simulink model "Geometric_DMP_R2022a"  (R2022a)
settings: Solver=FixedStepDiscrete  StartTime=0.0  StopTime=T  FixedStep=Ts  RelTol=1e-3
undefined symbols (not defined in the file): a, b, DiscIntNeverNeededParam, eta, gd, gr, Ts, yd
libraries: simulink x2
settings Model: Creator=giovanni  LastModifiedBy=giovanni

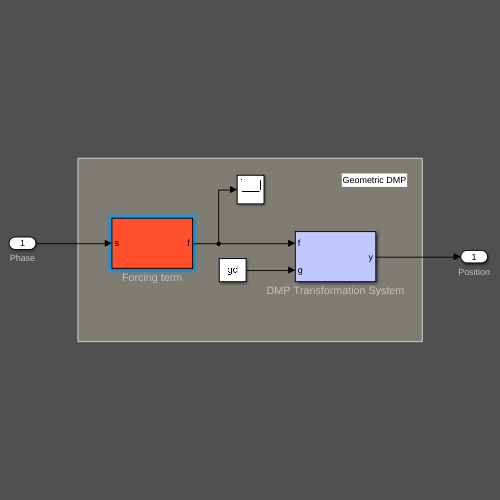
[thumbnail: Simulink's stored preview of the top-level diagram]
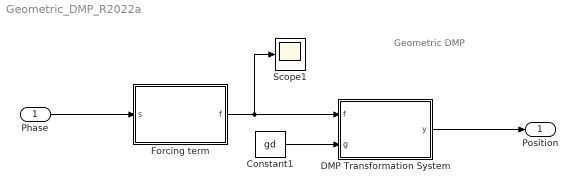
== system Geometric_DMP_R2022a ==
  note: Geometric DMP
  Phase : Inport
  Constant1 : Constant  Value=gd
  DMP Transformation System : Subsystem
  Forcing term : Subsystem
  Scope1 : Scope
  Position : Outport
  wires:
  Forcing term/1(f) -> Scope1/1, DMP Transformation System/1(f)
  Constant1/1 -> DMP Transformation System/2(g)
  DMP Transformation System/1(y) -> Position/1
  Phase/1 -> Forcing term/1(s)

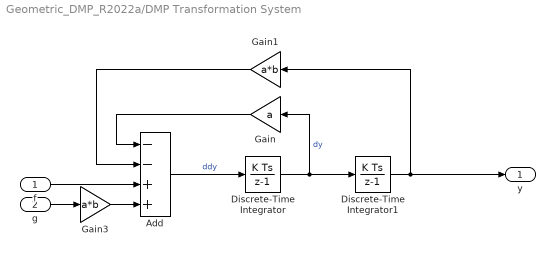
== system Geometric_DMP_R2022a/DMP Transformation System ==
  f : Inport
  g : Inport  Port=2
  Add : Sum  Inputs=--++
  Discrete-Time Integrator : DiscreteIntegrator  SampleTime=-1  ICPrevOutput=DiscIntNeverNeededParam  ICPrevScaledInput=DiscIntNeverNeededParam
  Discrete-Time Integrator1 : DiscreteIntegrator  InitialCondition=yd  SampleTime=-1  ICPrevOutput=DiscIntNeverNeededParam  ICPrevScaledInput=DiscIntNeverNeededParam
  Gain : Gain  Gain=a
  Gain1 : Gain  Gain=a*b
  Gain3 : Gain  Gain=a*b
  y : Outport
  wires:
  g/1 -> Gain3/1
  Discrete-Time Integrator/1 -> Gain/1, Discrete-Time Integrator1/1  "dy"
  Discrete-Time Integrator1/1 -> Gain1/1, y/1
  Add/1 -> Discrete-Time Integrator/1  "ddy"
  f/1 -> Add/3
  Gain/1 -> Add/1
  Gain1/1 -> Add/2
  Gain3/1 -> Add/4

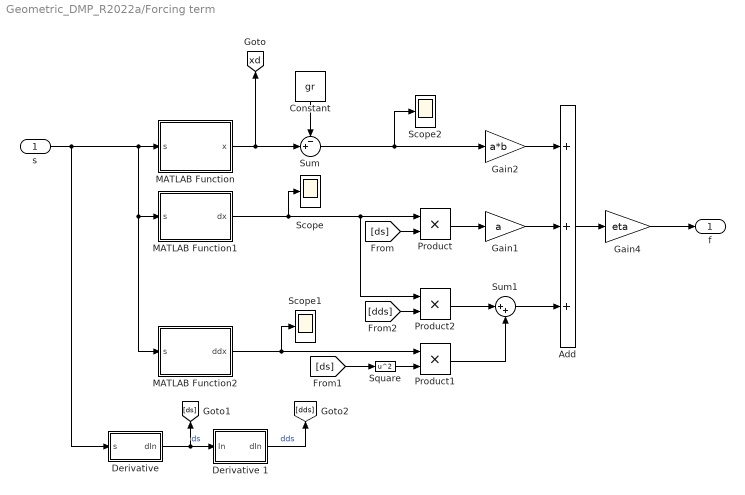
== system Geometric_DMP_R2022a/Forcing term ==
  s : Inport
  Add : Sum  Inputs=+++
  Constant : Constant  Value=gr
  "Derivative " : Subsystem
  Derivative 1 : Subsystem
  Gain1 : Gain  Gain=a
  Gain2 : Gain  Gain=a*b
  Gain4 : Gain  Gain=eta
  MATLAB Function : MATLAB Function  TreatAsAtomicUnit=on
  MATLAB Function1 : MATLAB Function  TreatAsAtomicUnit=on
  MATLAB Function2 : MATLAB Function  TreatAsAtomicUnit=on
  Product : Product
  Product1 : Product
  Product2 : Product
  Scope : Scope
  Scope1 : Scope
  Scope2 : Scope
  Square : Math  Operator=square
  Sum : Sum  Inputs=-+|
  Sum1 : Sum  Inputs=|++
  f : Outport
  tag scope: xd=global
  wires:
  s/1 -> "Derivative "/1(s), MATLAB Function2/1(s), MATLAB Function1/1(s), MATLAB Function/1(s)
  MATLAB Function/1(x) -> Sum/2, [xd]
  Constant/1 -> Sum/1
  MATLAB Function1/1(dx) -> Product2/1, Product/1, Scope/1
  Gain4/1 -> f/1
  Add/1 -> Gain4/1
  Sum/1 -> Scope2/1, Gain2/1
  Gain2/1 -> Add/1
  Gain1/1 -> Add/2
  MATLAB Function2/1(ddx) -> Scope1/1, Product1/1
  "Derivative "/1(dIn) -> [ds], Derivative 1/1(In)  "ds"
  Product/1 -> Gain1/1
  Derivative 1/1(dIn) -> [dds]  "dds"
  [ds] -> Product/2
  [ds] -> Square/1
  Square/1 -> Product1/2
  Sum1/1 -> Add/3
  Product1/1 -> Sum1/2
  Product2/1 -> Sum1/1
  [dds] -> Product2/2

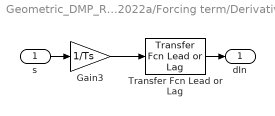
== system Geometric_DMP_R2022a/Forcing term/Derivative  ==
  s : Inport
  Gain3 : Gain  Gain=1/Ts
  Transfer Fcn Lead or Lag : simulink/Discrete/Transfer Fcn Lead or Lag  PoleZ=4.54e-05  ZeroZ=1.0  ICPrevOutput=0.0  ICPrevInput=0.0  DoSatur=off
      settings: SourceProductBaseCode=SL
  dIn : Outport
  wires:
  Gain3/1 -> Transfer Fcn Lead or Lag/1
  Transfer Fcn Lead or Lag/1 -> dIn/1
  s/1 -> Gain3/1

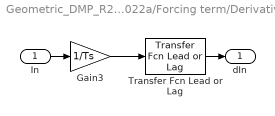
== system Geometric_DMP_R2022a/Forcing term/Derivative 1 ==
  In : Inport
  Gain3 : Gain  Gain=1/Ts
  Transfer Fcn Lead or Lag : simulink/Discrete/Transfer Fcn Lead or Lag  PoleZ=4.54e-05  ZeroZ=1.0  ICPrevOutput=0.0  ICPrevInput=0.0  DoSatur=off
      settings: SourceProductBaseCode=SL
  dIn : Outport
  wires:
  Gain3/1 -> Transfer Fcn Lead or Lag/1
  Transfer Fcn Lead or Lag/1 -> dIn/1
  In/1 -> Gain3/1

== matlab function Geometric_DMP_R2022a/Forcing term/MATLAB Function1 ==
  data: s input; dx output
function dx = dx_generator(s)

    dx = dx1_of_s(s);
    
end

== matlab function Geometric_DMP_R2022a/Forcing term/MATLAB Function2 ==
  data: s input; ddx output
function ddx = ddx_generator(s)

    ddx = ddx1_of_s(s);
    
end

== matlab function Geometric_DMP_R2022a/Forcing term/MATLAB Function ==
  data: s input; x output
function x = x_generator(s)

    x = x1_of_s(s);
    
end
